simulink model "PID_Model"  (Simulink 7.3)
settings: Solver=ode15s  StartTime=0.0  StopTime=20  RelTol=1e-6
undefined symbols (not defined in the file or in its folder): Kd, Ki, Kp
settings Model: Creator=tongji_HEV  LastModifiedBy=tongji_HEV
settings DataIOCC: SignalLoggingName=sigsOut
settings OptimizationCC: InitFltsAndDblsToZero=on
settings DebuggingCC: SaveWithParameterizedLinksMsg=none  SignalResolutionControl=TryResolveAllWithWarning  SolverPrmCheckMsg=none  MultiTaskDSMMsg=warning  MultiTaskCondExecSysMsg=none  StrictBusMsg=None
settings HardwareCC: TargetUnknown=on
settings RTWCC: IncludeERTFirstTime=on
settings GRTTargetCC: TargetFcnLib=ansi_tfl_tmw.mat

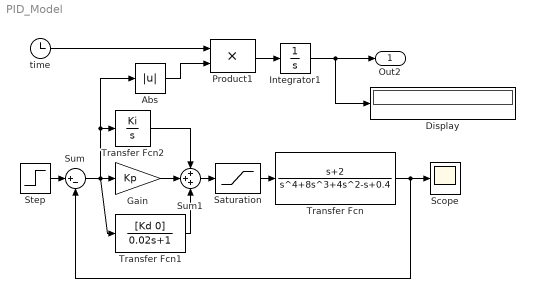
== system PID_Model ==
  Abs : Abs  ZeroCross=off  SaturateOnIntegerOverflow=on
  Display : Display
  Gain : Gain  Gain=Kp  ParameterDataType=sfix(16)  ParameterScaling=2^0  OutDataType=sfix(16)  OutScaling=2^0
  Integrator1 : Integrator
  Product1 : Product  OutDataType=sfix(16)  OutScaling=2^0  SaturateOnIntegerOverflow=on  OutDataTypeStr=Inherit: Same as first input
  Saturation : Saturate  UpperLimit=5  LowerLimit=-5
  Scope : Scope
      settings: TimeRange=10  YMin=0  YMax=1.4  SaveName=yy  DataFormat=Array
  Step : Step  Time=0  SampleTime=0
  Sum : Sum  Inputs=|+-  OutDataType=sfix(16)  OutScaling=2^0  SaturateOnIntegerOverflow=on
  Sum1 : Sum  Inputs=+++  OutDataType=sfix(16)  OutScaling=2^0  SaturateOnIntegerOverflow=on
  Transfer Fcn : TransferFcn  Numerator=[1 2 ]  Denominator=[1 8 4 -1 0.4]
  Transfer Fcn1 : TransferFcn  Numerator=[Kd 0]  Denominator=[0.02 1 ]
  Transfer Fcn2 : TransferFcn  Numerator=Ki  Denominator=[1 0 ]
  time : Clock
      settings: Decimation=10
  Out2 : Outport  OutDataType=sfix(16)  OutScaling=2^0
  wires:
  Step/1 -> Sum/1
  Sum/1 -> Transfer Fcn1/1, Gain/1, Abs/1, Transfer Fcn2/1
  Transfer Fcn/1 -> Scope/1, Sum/2
  time/1 -> Product1/1
  Integrator1/1 -> Out2/1, Display/1
  Product1/1 -> Integrator1/1
  Abs/1 -> Product1/2
  Sum1/1 -> Saturation/1
  Saturation/1 -> Transfer Fcn/1
  Gain/1 -> Sum1/2
  Transfer Fcn1/1 -> Sum1/3
  Transfer Fcn2/1 -> Sum1/1
